simulink model "SpringMassDamperModel"  (R2024b)
settings: Solver=VariableStepAuto  StartTime=0.0  StopTime=10.0  RelTol=1e-3

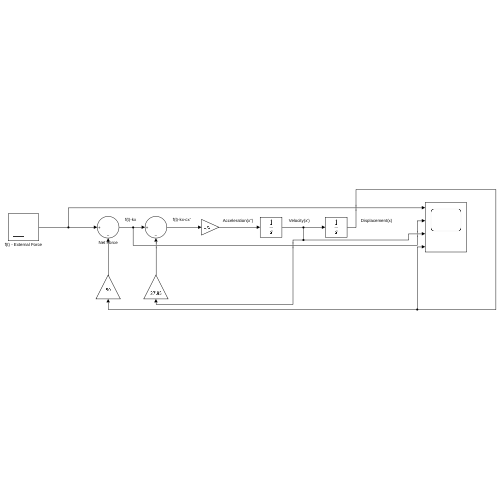
[thumbnail: Simulink's stored preview of the top-level diagram]
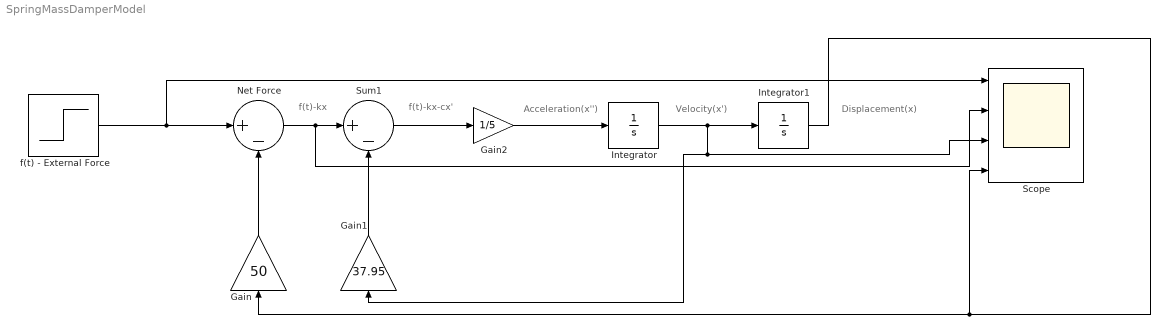
== system SpringMassDamperModel ==
  note: f(t)-kx-cx'
  note: f(t)-kx
  note: Acceleration(x'')
  note: Velocity(x')
  note: Displacement(x)
  Gain : Gain  Gain=50
  Gain1 : Gain  Gain=37.95
  Gain2 : Gain  Gain=1/5
  Integrator : Integrator
  Integrator1 : Integrator  InitialCondition=1
  Net Force : Sum  Inputs=|+-
  Scope : Scope  NumInputPorts=4
  Sum1 : Sum  Inputs=|+-
  f(t) - External Force : Step  After=5  SampleTime=0
  wires:
  Integrator1/1 -> Scope/4, Gain/1
  Integrator/1 -> Gain1/1, Scope/3, Integrator1/1
  Sum1/1 -> Gain2/1
  f(t) - External Force/1 -> Scope/1, Net Force/1
  Gain/1 -> Net Force/2
  Net Force/1 -> Scope/2, Sum1/1
  Gain2/1 -> Integrator/1
  Gain1/1 -> Sum1/2
